simulink model "controlPI_secador_solar"  (R2024b)
settings: Solver=VariableStepAuto  StartTime=0.0  StopTime=1000  RelTol=1e-3
values from neighbouring files (symbols this model uses):
  Kp = -0.00311    [tf2.mat]
  m_p_r = 0.02    [G.mat]
  To_r = 58.83    [G.mat]
undefined symbols (not defined in the file or in its folder): T_c, Ti
settings Model: Creator=Celso  LastModifiedBy=Salvador

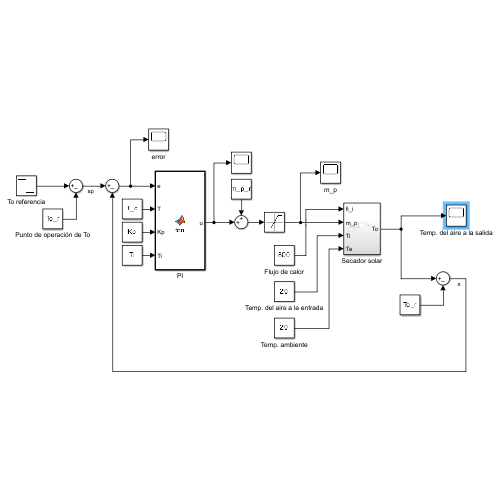
[thumbnail: Simulink's stored preview of the top-level diagram]
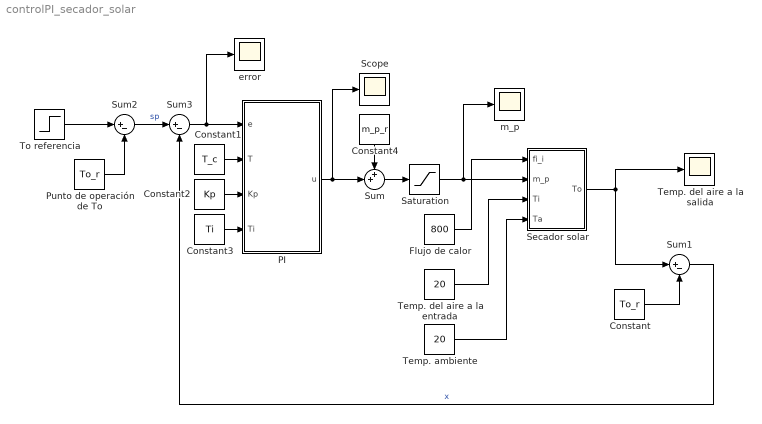
== system controlPI_secador_solar ==
  Constant : Constant  Value=To_r
  Constant1 : Constant  Value=T_c
  Constant2 : Constant  Value=Kp
  Constant3 : Constant  Value=Ti
  Constant4 : Constant  Value=m_p_r
  Flujo de calor : Constant  Value=800
  PI : MATLAB Function  TreatAsAtomicUnit=on  SystemSampleTime=T_c
  Punto de operación de To : Constant  Value=To_r
  Saturation : Saturate  UpperLimit=0.1  LowerLimit=0
  Scope : Scope
  Secador solar : Subsystem
  Sum : Sum  Inputs=++|
  Sum1 : Sum  Inputs=|+-
  Sum2 : Sum  Inputs=|+-
  Sum3 : Sum  Inputs=|+-
  Temp. ambiente : Constant  Value=20
  Temp. del aire a la entrada : Constant  Value=20
  Temp. del aire a la salida : Scope
  To referencia : Step  Time=500  Before=60  After=40  SampleTime=0
  error : Scope
  m_p : Scope
  wires:
  Temp. del aire a la entrada/1 -> Secador solar/3(Ti)
  Temp. ambiente/1 -> Secador solar/4(Ta)
  Secador solar/1(To) -> Sum1/1, Temp. del aire a la salida/1
  Flujo de calor/1 -> Secador solar/1(fi_i)
  Constant/1 -> Sum1/2
  To referencia/1 -> Sum2/1
  Punto de operación de To/1 -> Sum2/2
  Sum2/1 -> Sum3/1  "sp"
  Sum1/1 -> Sum3/2  "x"
  Sum3/1 -> error/1, PI/1(e)
  PI/1(u) -> Scope/1, Sum/2
  Constant4/1 -> Sum/1
  Sum/1 -> Saturation/1
  Constant1/1 -> PI/2(T)
  Constant2/1 -> PI/3(Kp)
  Constant3/1 -> PI/4(Ti)
  Saturation/1 -> m_p/1, Secador solar/2(m_p)

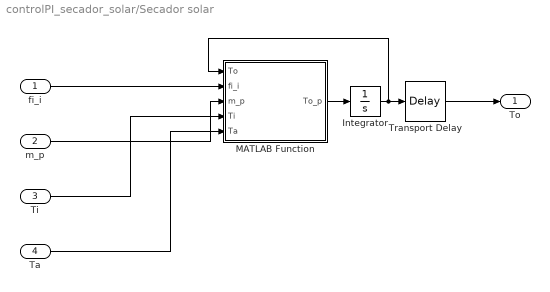
== system controlPI_secador_solar/Secador solar ==
  fi_i : Inport
  m_p : Inport  Port=2
  Ti : Inport  Port=3
  Ta : Inport  Port=4
  Integrator : Integrator  InitialCondition=20
  MATLAB Function : MATLAB Function  TreatAsAtomicUnit=on
  Transport Delay : TransportDelay  DelayTime=10  InitialOutput=20
  To : Outport
  wires:
  Integrator/1 -> MATLAB Function/1(To), Transport Delay/1
  MATLAB Function/1(To_p) -> Integrator/1
  fi_i/1 -> MATLAB Function/2(fi_i)
  Ta/1 -> MATLAB Function/5(Ta)
  Ti/1 -> MATLAB Function/4(Ti)
  m_p/1 -> MATLAB Function/3(m_p)
  Transport Delay/1 -> To/1

== matlab function controlPI_secador_solar/PI ==
  data: e input; T input; u output; Kp input; Ti input
function u = fcn(e,T, Kp, Ti)

persistent I_ant;

if isempty(I_ant),
    I_ant=0;
end;

I = I_ant + e*T;
u = Kp*(e+ (1/Ti)*I);

I_ant = I;

== matlab function controlPI_secador_solar/Secador solar/MATLAB Function ==
  data: To input; To_p output; fi_i input; m_p input; Ti input; Ta input
function To_p = fcn(To,fi_i,m_p,Ti,Ta)

%Simula el calentamiento del aire en un secador solar
%To: temperatura del aire a la salida (°C)
%Ti: temperatura del aire a la entrada (°C)
%V: voltaje aplicado a la resistencia
%   eléctrica del calentador (volt)
%m_p: flujo de masa del aire que ingresa y sale del
%     secador solar (Kg/seg)
%Ta: temperatura ambiente (°C)

M = 0.9; %masa del aire en el secador solar (Kg)
c = 1005; %calor específico del aire (J/Kg-°C)
%fi_i = 800; %Flujo de calor proporcionada por la radiación solar
R = 2; %Resistencia térmica (°C.seg/J)


To_p = fi_i/(M*c) - m_p*(To-Ti)/M - (To-Ta)/(M*c*R)
